simulink model "Phase_Jump_A_B_A"  (Simulink 9.2)
settings: Solver=ode4  StartTime=0.0  StopTime=101.5  FixedStep=Ts  RelTol=1e-3  EnableMultiTasking=on
PreLoadFcn:
  | Ts=40e-6;Core_Num = 0;
PostLoadFcn:
  | Ts=40e-6;Core_Num = 0;
InitFcn:
  | Ts=40e-6;Core_Num = 0;
libraries: rtio_opalrt_ml605ex1 x4, rtlab x3, artemis x1, powerlib x1
settings Model: ARTEMISmethode_block_infos=$$__separator__$$Phase_Jump_A_B_A/ARTEMIS Guide1$$__separator__$$  Creator=DETLDAQ  LastModifiedBy=DETLDAQ
settings OptimizationCC: BlockReduction=off  BooleanDataType=off  OptimizeBlockIOStorage=off  BufferReuse=off  GlobalBufferReuse=off  ExpressionFolding=off  LocalBlockOutputs=off  OptimizeDataStoreBuffers=off  BusAssignmentInplaceUpdate=off
settings DebuggingCC: SaveWithParameterizedLinksMsg=none  SignalResolutionControl=TryResolveAllWithWarning  MultiTaskDSMMsg=warning  MultiTaskCondExecSysMsg=none  FcnCallInpInsideContextMsg=error
settings HardwareCC: TargetUnknown=on
settings GRTTargetCC: CombineOutputUpdateFcns=on  GRTInterface=off
settings SimscapeCC: SimscapeNormalizeSystem=off

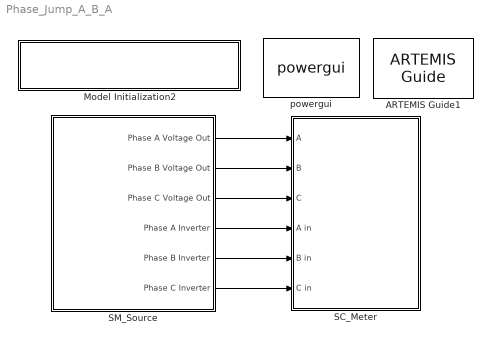
== system Phase_Jump_A_B_A ==
  ARTEMIS Guide1 : artemis/ARTEMIS/ARTEMIS Guide  Tag=FTSSmethode_opal_4hx0r99  Description=5.0_z1  lock=on  Ts=Ts  ssn=on  opt=art5  dyna=off  nb_perm=4  RT_fullcomp=off  ssn_itvc=off  ssn_ivic=off  ssn_ext=off  ssn_solver=Backward Euler  iter_type=iSWITCH and iMOV only (default)  ssn_ImpulseLoopBlockedStateUpdate=5  ssn_mov_iter_number=5  ssn_switch_iter_number=5  ssn_lu_or_ldlt=LU (more robust)  ssn_nib_type_verify=on  ssn_use_lu=on  ssn_use_ldlt=off  ssn_impulse=on  ssn_quasimpulse=off  ssn_impulse_loop=5  paraExtinctionThy=off  Thy_Impulse=off  dtc=Off  dtc_opt=normal  ao=on  simtype=off  ct_mac=off  lin_mov=off  lsp=[0.001 2]  spike_skip=Disabled  dtc_extra=1  dtc_sws=normal  dtc_pied=0.5  SPSRulesBlock=SPSRules  tre=off  ctmm=off  LF=on  dpl_type=ARTEMiS DPL  rlc_type=off  custom_type=off  para=on  ssn_full_iteration=off
  Model Initialization2 : Subsystem  AncestorBlock=artemis/Tools /Misc/Model Initialization  mask(Model Functions){InitFcnX=Ts=40e-6;Core_Num = 0;, prel=on, posl=on, inif=on, strf=off}
      mask prompts: InitFcnX "Initialisation"; prel "Preload Function"; posl "PostLoad Function"; inif "InitFcn"; strf "StartFcn"
      mask init:
      | currentBlock = gcb;
      | root = bdroot(currentBlock);
      | 
      | if ~strcmp(get_param(root,'BlockDiagramType'),'library')
      |     if prel==1
      |         set_param(root, 'PreLoadFcn', InitFcnX);
      |     else
      |         set_param(root, 'PreLoadFcn', '');
      |     end
      |     if inif==1
      |         set_param(root, 'InitFcn', InitFcnX);
      |     else
      |         set_param(root, 'InitFcn', '');
      |     end
      |     if strf==1
      |         set_param(root, 'StartFcn', InitFcnX);
      |     else
      |         set_param(root, 'StartFcn', '');
      |     end
      |     if posl==1
      |         set_param(root, 'PostLoadFcn', InitFcnX);
      |     else
      |         set_param(root, 'PostLoadFcn', '');
      |     end
      | end
      | 
      | pos = get_param(currentBlock, 'Position');
      | width = pos(3) - pos(1); height = pos(4) - pos(2);
      | txt = [ upper(root) '\n' '- InitFcn. . . . . '  get_param(root, 'InitFcn') ];
      settings: CopyFcn=set_param(gcb,'LinkStatus','inactive')
      mask Display: text(5, height*0.5, txt, 'horizontalAlignment', 'left', 'verticalAlignment', 'middle') ;
  SC_Meter : Subsystem
  SM_Source : Subsystem
  powergui : powerlib/powergui  Priority=1  SimulationMode=Discrete  SampleTime=Ts  frequency=60  Iterations=50  frequencyindice=0  Pbase=100e6  ErrMax=1e-4  UnitsV=kV  UnitsW=MW  buscounter=0  FunctionMessages=off  echomessages=off  EnableUseOfTLC=off  CurrentSourceSwitches=off  DisableSnubberDevices=off  DisableRonSwitches=off  DisableVfSwitches=off  DisplayEquations=off  SolverType=Backward Euler  Interpol=off  ExternalGateDelay=off  methode=off  Ts=100  x0status=blocks  SPID=off  SwTol=0  HookPort=off  RestoreLinks=warning  ResistiveCurrentMeasurement=off  Frange=[0:2:500]  Ylog=off  Xlog=on  ShowGrid=off  save=off  variable=ZData  structure=0  ZoomFFT=off  StartTime=0.0  cycles=1  DisplayStyle=1  fundamental=60  FreqAxis=off  MaxFrequency=1000  frequencyindicesteady=1  RmsSteady=1  display=off
  wires:
  SM_Source/5(Phase B Inverter) -> SC_Meter/5(B in)
  SM_Source/6(Phase C Inverter) -> SC_Meter/6(C in)
  SM_Source/4(Phase A Inverter) -> SC_Meter/4(A in)
  SM_Source/2(Phase B Voltage Out) -> SC_Meter/2(B)
  SM_Source/1(Phase A Voltage Out) -> SC_Meter/1(A)
  SM_Source/3(Phase C Voltage Out) -> SC_Meter/3(C)

== system Phase_Jump_A_B_A/Model Initialization2 ==

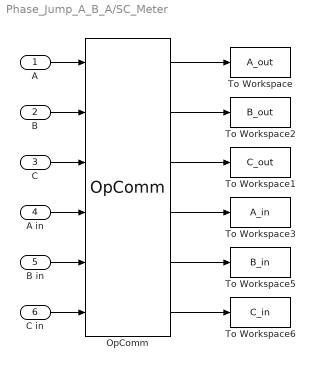
== system Phase_Jump_A_B_A/SC_Meter ==
  A : Inport
  B : Inport  Port=2
  C : Inport  Port=3
  A in : Inport  Port=4
  B in : Inport  Port=5
  C in : Inport  Port=6
  OpComm : rtlab/OpComm  nbport=6  groupe_acq=1  subsys_rate=Ts  st=0  Synchronization=on  Interpolation=on  Threshold=1.0  Missed_Data=off  Sim_Time=off  Samples=off  dynSigOut=off  from_console=0  warning_done=off  writeOpCommFile=off  Offset=off
  To Workspace : ToWorkspace  VariableName=A_out  SaveFormat=Timeseries  SampleTime=Ts
  To Workspace1 : ToWorkspace  VariableName=C_out  SaveFormat=Timeseries  SampleTime=Ts
  To Workspace2 : ToWorkspace  VariableName=B_out  SaveFormat=Timeseries  SampleTime=Ts
  To Workspace3 : ToWorkspace  VariableName=A_in  SaveFormat=Timeseries  SampleTime=Ts
  To Workspace5 : ToWorkspace  VariableName=B_in  SaveFormat=Timeseries  SampleTime=Ts
  To Workspace6 : ToWorkspace  VariableName=C_in  SaveFormat=Timeseries  SampleTime=Ts
  wires:
  OpComm/1 -> To Workspace/1
  OpComm/3 -> To Workspace1/1
  OpComm/2 -> To Workspace2/1
  A/1 -> OpComm/1
  B/1 -> OpComm/2
  C/1 -> OpComm/3
  OpComm/4 -> To Workspace3/1
  OpComm/5 -> To Workspace5/1
  OpComm/6 -> To Workspace6/1
  A in/1 -> OpComm/4
  B in/1 -> OpComm/5
  C in/1 -> OpComm/6

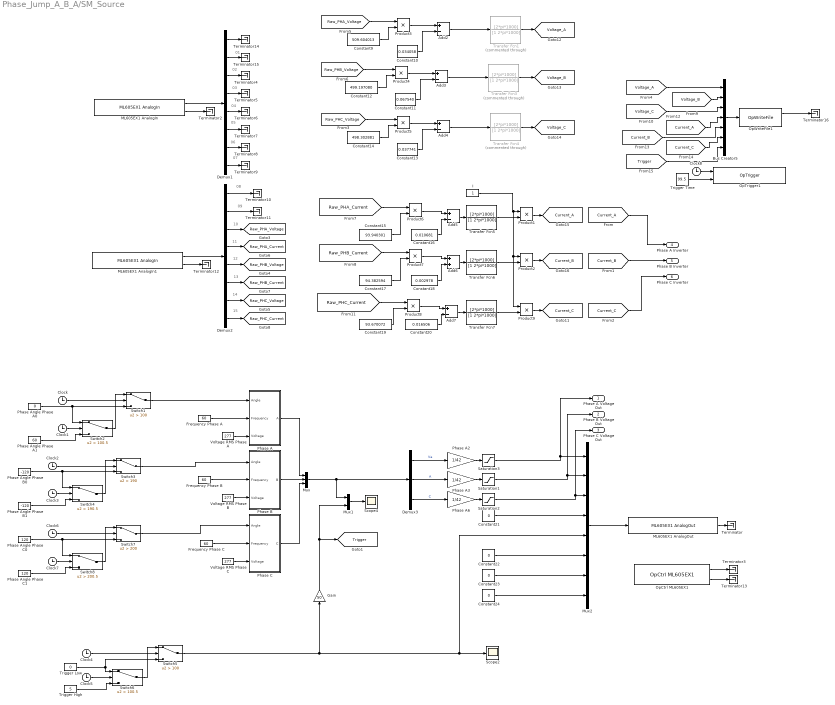
== system Phase_Jump_A_B_A/SM_Source ==
  note: 15
  note: 14
  note: 13
  note: 12
  note: 11
  note: 10
  note: 09
  note: 08
  note: 07
  note: 06
  note: 05
  note: 04
  note: 03
  note: 02
  note: 01
  Add{2..5,7} (5 alike) : Sum  Inputs=+-
  Add6 : Sum
  Bus Creator5 : BusCreator  Inputs=7
  Clock{,1..8} (9 alike) : Clock
      Clock settings: Decimation=30
      Clock1 settings: Decimation=30
      Clock2 settings: Decimation=30
      Clock3 settings: Decimation=30
      Clock4 settings: Decimation=30
      Clock5 settings: Decimation=30
      Clock6 settings: Decimation=30
      Clock7 settings: Decimation=30
  Constant10 : Constant  Value=0.034058
  Constant11 : Constant  Value=0.067540
  Constant12 : Constant  Value=499.197080
  Constant13 : Constant  Value=0.037741
  Constant14 : Constant  Value=498.302881
  Constant15 : Constant  Value=93.940301
  Constant16 : Constant  Value=0.010681
  Constant17 : Constant  Value=94.382594
  Constant18 : Constant  Value=0.002978
  Constant19 : Constant  Value=93.670072
  Constant20 : Constant  Value=0.016506
  Constant{21..24} (4 alike) : Constant  Value=0
  Constant9 : Constant  Value=509.604013
  Demux1 : Demux  Outputs=8
  Demux2 : Demux  Outputs=8
  Demux3 : Demux  Outputs=3
  Frequency Phase A : Constant  Value=60
  Frequency Phase B : Constant  Value=60
  Frequency Phase C : Constant  Value=60
  Gain : Gain  Gain=50
  I : Constant
  ML605EX1 AnalogIn : rtio_opalrt_ml605ex1/ML605EX1 AnalogIn  CtrlName='ML605EX1 Ctrl'  portNb=1  FcnNos=Slot 1 Module B Subsection 1  size=16  maxcount=8  count=8  numchan=8  sampleTime=0
      settings: AttributesFormatString=%<CtrlName>
  ML605EX1 AnalogIn1 : rtio_opalrt_ml605ex1/ML605EX1 AnalogIn  CtrlName='ML605EX1 Ctrl'  portNb=2  FcnNos=Slot 1 Module B Subsection 2  size=16  maxcount=8  count=8  numchan=8  sampleTime=0
      settings: AttributesFormatString=%<CtrlName>
  ML605EX1 AnalogOut : rtio_opalrt_ml605ex1/ML605EX1 AnalogOut  CtrlName='ML605EX1 Ctrl'  portNb=1  FcnNos=Slot 1 Module A Subsection 1  size=16  maxcount=8  count=8  numchan=8  israngeinput=off  voltagerange=[-16 ... 16]  slot=0  side=0  mismatch=0  slotside=Slot_1_Module_A
      settings: AttributesFormatString=%<CtrlName>
  Mux : Mux  Inputs=3
  Mux1 : Mux  Inputs=2
  Mux2 : Mux  Inputs=8
  OpCtrl ML605EX1 : rtio_opalrt_ml605ex1/OpCtrl ML605EX1  CtrlName='ML605EX1 Ctrl'  boardid=0  BitstreamFilename=ML605_2-EX-0029-2_2_6_61-32Aio_32DioSelectable-01-01.bin  numconfig=-1  mode=Master  externalClock=off  decimRtsi=0  calibIO=off  SampleTime=0  loadinport=-1
  OpTrigger1 : rtlab/DataLogging/OpTrigger  Trig_Type=TRIGGER SIGNAL >= TRIGGER LEVEL  Trig_Offset=0  Acq_Group=29
  OpWriteFile1 : rtlab/DataLogging/OpWriteFile  Static_File=on  varname=Data  Filename=SVP_Data.mat  rtpath=''  nrtpath=''  Acq_Group=29  file_size=1e+10  write_offline=off  Sim_Mode=off  Nb_Samples=1000  Buffer_size=1000000
  Phase A : Subsystem
  Phase A2 : Gain  Gain=1/42
  Phase A3 : Gain  Gain=1/42
  Phase A6 : Gain  Gain=1/42
  Phase Angle Phase A0 : Constant  Value=0
  Phase Angle Phase A1 : Constant  Value=60
  Phase Angle Phase B0 : Constant  Value=-120
  Phase Angle Phase B1 : Constant  Value=-120
  Phase Angle Phase C0 : Constant  Value=120
  Phase Angle Phase C1 : Constant  Value=120
  Phase B : Subsystem
  Phase C : Subsystem
  Product{1..9} (9 alike) : Product
  Saturation1 : Saturate  UpperLimit=11  LowerLimit=-11
  Saturation2 : Saturate  UpperLimit=11  LowerLimit=-11
  Saturation3 : Saturate  UpperLimit=11  LowerLimit=-11
  Scope2 : Scope
  Scope4 : Scope
  Switch1 : Switch  Criteria=u2 > Threshold  Threshold=100
  Switch2 : Switch  Criteria=u2 > Threshold  Threshold=100.5
  Switch3 : Switch  Criteria=u2 > Threshold  Threshold=190
  Switch4 : Switch  Criteria=u2 > Threshold  Threshold=190.5
  Switch5 : Switch  Criteria=u2 > Threshold  Threshold=100
  Switch6 : Switch  Criteria=u2 > Threshold  Threshold=100.5
  Switch7 : Switch  Criteria=u2 > Threshold  Threshold=200
  Switch8 : Switch  Criteria=u2 > Threshold  Threshold=200.5
  Terminator{,2..16} (16 alike) : Terminator
  Transfer Fcn1 : TransferFcn  Commented=through  Numerator=[2*pi*1000]  Denominator=[1 2*pi*1000]
  Transfer Fcn3 : TransferFcn  Commented=through  Numerator=[2*pi*1000]  Denominator=[1 2*pi*1000]
  Transfer Fcn4 : TransferFcn  Commented=through  Numerator=[2*pi*1000]  Denominator=[1 2*pi*1000]
  Transfer Fcn5 : TransferFcn  Numerator=[2*pi*1000]  Denominator=[1 2*pi*1000]
  Transfer Fcn6 : TransferFcn  Numerator=[2*pi*1000]  Denominator=[1 2*pi*1000]
  Transfer Fcn7 : TransferFcn  Numerator=[2*pi*1000]  Denominator=[1 2*pi*1000]
  Trigger High : Constant  Value=5
  Trigger Low : Constant  Value=0
  Trigger Time : Constant  Value=99.5
  Voltage RMS Phase A : Constant  Value=277
  Voltage RMS Phase B : Constant  Value=277
  Voltage RMS Phase C : Constant  Value=277
  Phase A Voltage Out : Outport
  Phase B Voltage Out : Outport  Port=2
  Phase C Voltage Out : Outport  Port=3
  Phase A Inverter : Outport  Port=4
  Phase B Inverter : Outport  Port=5
  Phase C Inverter : Outport  Port=6
  tag scope: Current_A=global, Current_B=global, Current_C=global, Raw_PHA_Current=global, Raw_PHA_Voltage=global, Raw_PHB_Current=global, Raw_PHB_Voltage=global, Raw_PHC_Current=global, Raw_PHC_Voltage=global, Trigger=global, Voltage_A=global, Voltage_B=global, Voltage_C=global
  wires:
  Frequency Phase A/1 -> Phase A/2(Frequency)
  Voltage RMS Phase A/1 -> Phase A/3(Voltage)
  Phase A/1(A) -> Mux/1
  Frequency Phase B/1 -> Phase B/2(Frequency)
  Voltage RMS Phase B/1 -> Phase B/3(Voltage)
  Phase B/1(B) -> Mux/2
  Frequency Phase C/1 -> Phase C/2(Frequency)
  Voltage RMS Phase C/1 -> Phase C/3(Voltage)
  Phase C/1(C) -> Mux/3
  Clock/1 -> Switch1/2
  Clock1/1 -> Switch2/2
  Switch2/1 -> Switch1/1
  Phase Angle Phase A1/1 -> Switch2/3
  Phase Angle Phase A0/1 -> Switch2/1, Switch1/3
  Demux1/3 -> Terminator4/1
  Demux1/4 -> Terminator5/1
  Demux1/5 -> Terminator6/1
  Demux1/6 -> Terminator7/1
  Demux1/7 -> Terminator8/1
  Demux1/8 -> Terminator9/1
  Demux2/3 -> [Raw_PHA_Voltage]
  Demux2/1 -> Terminator10/1
  Demux2/2 -> Terminator11/1
  ML605EX1 AnalogIn/1 -> Demux1/1
  ML605EX1 AnalogIn/2 -> Terminator2/1
  ML605EX1 AnalogIn1/1 -> Demux2/1
  ML605EX1 AnalogIn1/2 -> Terminator12/1
  Demux1/1 -> Terminator14/1
  Demux1/2 -> Terminator15/1
  Demux2/4 -> [Raw_PHA_Current]
  Demux2/5 -> [Raw_PHB_Voltage]
  Demux2/6 -> [Raw_PHB_Current]
  Demux2/7 -> [Raw_PHC_Voltage]
  Demux2/8 -> [Raw_PHC_Current]
  Constant10/1 -> Add2/2
  Constant9/1 -> Product3/2
  Add2/1 -> Transfer Fcn1/1
  Product4/1 -> Add3/1
  Constant11/1 -> Add3/2
  Constant12/1 -> Product4/2
  Add3/1 -> Transfer Fcn3/1
  Product5/1 -> Add4/1
  Constant13/1 -> Add4/2
  Constant14/1 -> Product5/2
  Add4/1 -> Transfer Fcn4/1
  [Raw_PHB_Voltage] -> Product4/1
  [Raw_PHC_Voltage] -> Product5/1
  Constant15/1 -> Product6/2
  Constant16/1 -> Add5/2
  Product6/1 -> Add5/1
  [Raw_PHA_Current] -> Product6/1
  Add5/1 -> Transfer Fcn5/1
  Constant17/1 -> Product7/2
  Constant18/1 -> Add6/2
  Product7/1 -> Add6/1
  [Raw_PHB_Current] -> Product7/1
  Add6/1 -> Transfer Fcn6/1
  Product8/1 -> Add7/1
  [Raw_PHC_Current] -> Product8/1
  Add7/1 -> Transfer Fcn7/1
  Transfer Fcn5/1 -> Product1/2
  Transfer Fcn7/1 -> Product9/2
  Transfer Fcn6/1 -> Product2/2
  Transfer Fcn4/1 -> [Voltage_C]
  Transfer Fcn3/1 -> [Voltage_B]
  Transfer Fcn1/1 -> [Voltage_A]
  Product1/1 -> [Current_A]
  Product2/1 -> [Current_B]
  Product9/1 -> [Current_C]
  I/1 -> Product9/1, Product2/1, Product1/1
  Constant19/1 -> Product8/2
  Constant20/1 -> Add7/2
  Constant24/1 -> Mux2/8
  Constant23/1 -> Mux2/7
  Constant22/1 -> Mux2/6
  Constant21/1 -> Mux2/4
  Switch5/1 -> Gain/1, Scope2/1, Mux2/5
  Mux2/1 -> ML605EX1 AnalogOut/1
  Demux3/1 -> Phase A2/1  "Va"
  Mux/1 -> Mux1/1, Demux3/1
  OpCtrl ML605EX1/1 -> Terminator3/1
  OpCtrl ML605EX1/2 -> Terminator13/1
  ML605EX1 AnalogOut/1 -> Terminator/1
  Phase A3/1 -> Saturation1/1
  Phase A6/1 -> Saturation2/1
  Saturation3/1 -> Phase A Voltage Out/1, Mux2/1
  Saturation2/1 -> Phase C Voltage Out/1, Mux2/3
  Saturation1/1 -> Phase B Voltage Out/1, Mux2/2
  Demux3/3 -> Phase A6/1  "C"
  Phase A2/1 -> Saturation3/1
  Demux3/2 -> Phase A3/1  "A"
  [Raw_PHA_Voltage] -> Product3/1
  Product3/1 -> Add2/1
  [Current_B] -> Phase B Inverter/1
  [Current_A] -> Phase A Inverter/1
  [Current_C] -> Phase C Inverter/1
  Clock5/1 -> Switch6/2
  Trigger High/1 -> Switch6/3
  Switch6/1 -> Switch5/1
  Trigger Low/1 -> Switch5/3, Switch6/1
  Mux1/1 -> Scope4/1
  Gain/1 -> Mux1/2, [Trigger]
  Clock4/1 -> Switch5/2
  Switch7/1 -> Phase C/1(Angle)
  Switch1/1 -> Phase A/1(Angle)
  Switch3/1 -> Phase B/1(Angle)
  [Current_C] -> Bus Creator5/6
  Trigger Time/1 -> OpTrigger1/2
  [Current_A] -> Bus Creator5/4
  OpWriteFile1/1 -> Terminator16/1
  [Voltage_B] -> Bus Creator5/2
  Bus Creator5/1 -> OpWriteFile1/1
  Clock8/1 -> OpTrigger1/1
  [Voltage_C] -> Bus Creator5/3
  [Voltage_A] -> Bus Creator5/1
  [Current_B] -> Bus Creator5/5
  Clock2/1 -> Switch3/2
  Phase Angle Phase B1/1 -> Switch4/3
  Switch4/1 -> Switch3/1
  Clock3/1 -> Switch4/2
  Phase Angle Phase B0/1 -> Switch4/1, Switch3/3
  Phase Angle Phase C0/1 -> Switch8/1, Switch7/3
  Clock7/1 -> Switch8/2
  Phase Angle Phase C1/1 -> Switch8/3
  Clock6/1 -> Switch7/2
  Switch8/1 -> Switch7/1
  [Trigger] -> Bus Creator5/7

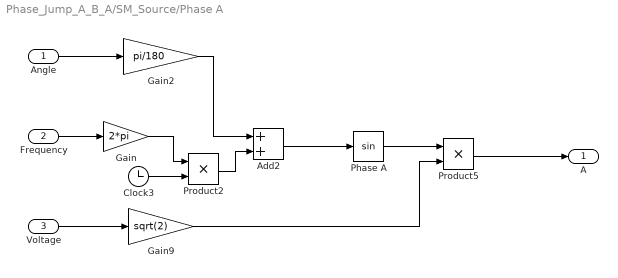
== system Phase_Jump_A_B_A/SM_Source/Phase A ==
  Angle : Inport
  Frequency : Inport  Port=2
  Voltage : Inport  Port=3
  Add2 : Sum
  Clock3 : Clock
  Gain : Gain  Gain=2*pi
  Gain2 : Gain  Gain=pi/180
  Gain9 : Gain  Gain=sqrt(2)
  Phase A : Trigonometry
  Product2 : Product
  Product5 : Product
  A : Outport
  wires:
  Phase A/1 -> Product5/1
  Gain2/1 -> Add2/1
  Voltage/1 -> Gain9/1
  Gain9/1 -> Product5/2
  Product2/1 -> Add2/2
  Clock3/1 -> Product2/2
  Frequency/1 -> Gain/1
  Angle/1 -> Gain2/1
  Add2/1 -> Phase A/1
  Gain/1 -> Product2/1
  Product5/1 -> A/1

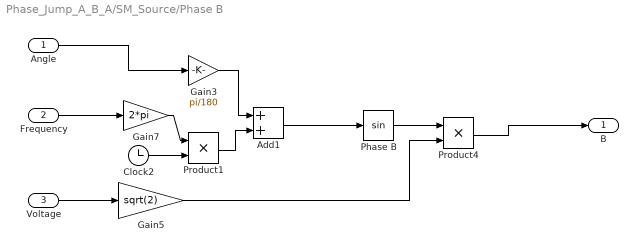
== system Phase_Jump_A_B_A/SM_Source/Phase B ==
  Angle : Inport
  Frequency : Inport  Port=2
  Voltage : Inport  Port=3
  Add1 : Sum
  Clock2 : Clock
  Gain3 : Gain  Gain=pi/180
  Gain5 : Gain  Gain=sqrt(2)
  Gain7 : Gain  Gain=2*pi
  Phase B : Trigonometry
  Product1 : Product
  Product4 : Product
  B : Outport
  wires:
  Phase B/1 -> Product4/1
  Gain3/1 -> Add1/1
  Product4/1 -> B/1
  Gain7/1 -> Product1/1
  Add1/1 -> Phase B/1
  Angle/1 -> Gain3/1
  Product1/1 -> Add1/2
  Clock2/1 -> Product1/2
  Frequency/1 -> Gain7/1
  Gain5/1 -> Product4/2
  Voltage/1 -> Gain5/1

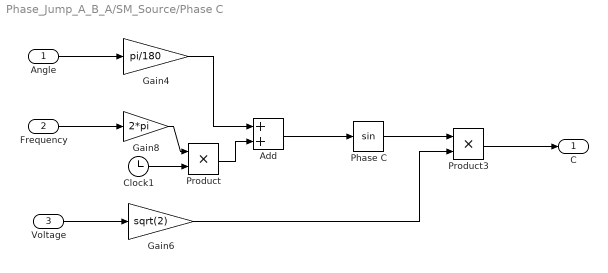
== system Phase_Jump_A_B_A/SM_Source/Phase C ==
  Angle : Inport
  Frequency : Inport  Port=2
  Voltage : Inport  Port=3
  Add : Sum
  Clock1 : Clock
  Gain4 : Gain  Gain=pi/180
  Gain6 : Gain  Gain=sqrt(2)
  Gain8 : Gain  Gain=2*pi
  Phase C : Trigonometry
  Product : Product
  Product3 : Product
  C : Outport
  wires:
  Clock1/1 -> Product/2
  Gain8/1 -> Product/1
  Phase C/1 -> Product3/1
  Frequency/1 -> Gain8/1
  Gain4/1 -> Add/1
  Product3/1 -> C/1
  Product/1 -> Add/2
  Add/1 -> Phase C/1
  Angle/1 -> Gain4/1
  Gain6/1 -> Product3/2
  Voltage/1 -> Gain6/1
